simulink subsystem "PEC_LQR"  (R2024a)
settings: Solver=VariableStepAuto  StartTime=0.0  StopTime=10.0  RelTol=1e-3
undefined symbols (not defined in the file): Sim, vehicle
settings Model: Creator=gurt1  LastModifiedBy=gurt1

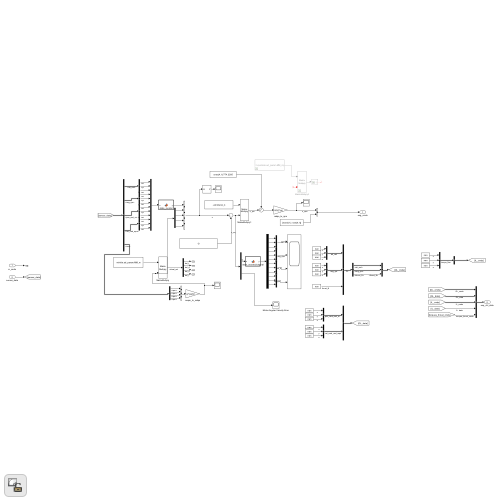
[thumbnail: Simulink's stored preview of the top-level diagram]
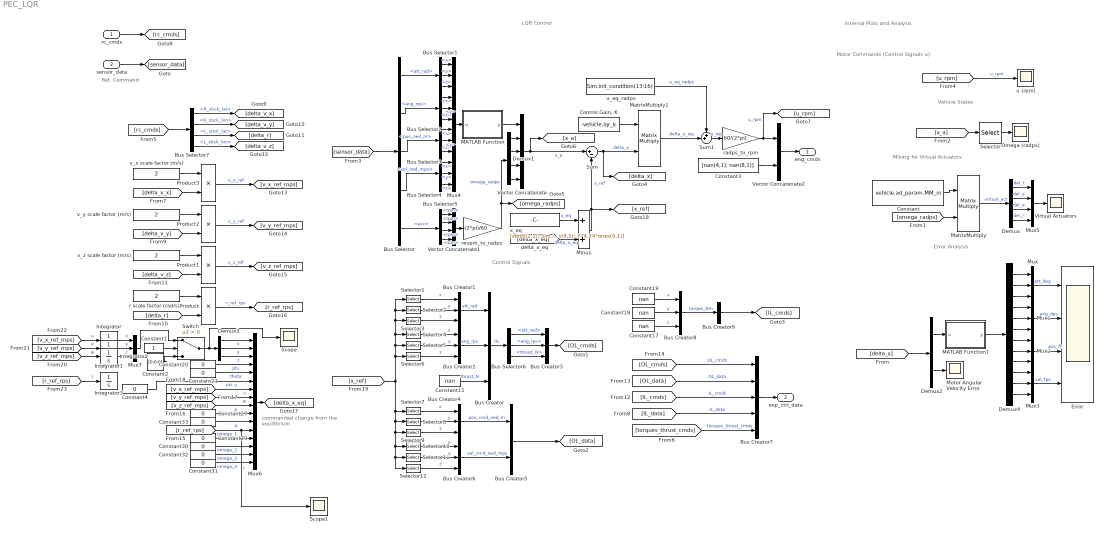
== system PEC_LQR ==
  note: commanded change from the equilibrium
  note: Control Signals
  note: Mixing for Virtual Actuators
  note: Error Analysis
  note: LQR Control
  note: Internal Plots and Analysis
  note: Vehicle States
  note: Motor Commands (Control Signals u)
  note: Ref. Command
  rc_cmds : Inport
  sensor_data : Inport  Port=2
  Bus Creator{,1..4,6,8} (7 alike) : BusCreator  Inputs=3
  Bus Creator5 : BusCreator  Inputs=2
  Bus Creator7 : BusCreator  Inputs=5
  Bus Creator9 : BusCreator  Inputs=1
  Bus Selector : BusSelector  OutputSignals=att_rad,ang_rps,pos_ned_m,vel_ned_mps,esc
  Bus Selector{1..4} (4 alike) : BusSelector  OutputSignals=x,y,z
  Bus Selector5 : BusSelector  OutputSignals=1.rpm,2.rpm,3.rpm,4.rpm
  Bus Selector6 : BusSelector  OutputSignals=att_rad,ang_rps,thrust_N
  Bus Selector7 : BusSelector  OutputSignals=sticks.R_stick_lat,sticks.R_stick_lon,sticks.L_stick_lat,sticks.L_stick_lon
  Constant : Constant  Value=vehicle.ad_param.MM_m
  Constant1 : Constant
  Constant{11,17..19} (4 alike) : Constant  Value=nan
  Constant2 : Constant  Value=[0;0;0]
  Constant{4,20..21,27,29..33} (9 alike) : Constant  Value=0
  Constant3 : Constant  Value=[nan(4,1); nan(8,1)]
  "Control Gain, K" : Constant  Value=-vehicle.lqr_k
  Demux : Demux
  Demux1 : Demux
  Demux2 : Demux  Outputs=[12 4]
  Demux3 : Demux  Outputs=3
  Demux4 : Demux  Outputs=12
  Error : Scope  NumInputPorts=4
  Integrator{,1..3} (4 alike) : Integrator
  MATLAB Function : MATLAB Function  TreatAsAtomicUnit=on
  MATLAB Function1 : MATLAB Function  TreatAsAtomicUnit=on
  MatrixMultiply : Product  Multiplication=Matrix(*)
  MatrixMultiply1 : Product  Multiplication=Matrix(*)
  Minus : Sum
  Motor Angular Velocity Error : Scope
  Mux{,1..3,7} (5 alike) : Mux  Inputs=3
  Mux4 : Mux  Inputs=12
  Mux5 : Mux
  Mux6 : Mux  Inputs=16
  Omega (radps) : Scope
  Product{,1..3} (4 alike) : Product
  Scope : Scope
  Scope1 : Scope
  Selector : Selector  InputPortWidth=16  IndexOptions=Index vector (dialog)  Indices=13:16  OutputSizes=1
  Selector1 : Selector  InputPortWidth=16  IndexOptions=Index vector (dialog)  Indices=4  OutputSizes=1
  Selector10 : Selector  InputPortWidth=16  IndexOptions=Index vector (dialog)  Indices=7  OutputSizes=1
  Selector11 : Selector  InputPortWidth=16  IndexOptions=Index vector (dialog)  Indices=8  OutputSizes=1
  Selector12 : Selector  InputPortWidth=16  IndexOptions=Index vector (dialog)  Indices=9  OutputSizes=1
  Selector2 : Selector  InputPortWidth=16  IndexOptions=Index vector (dialog)  Indices=5  OutputSizes=1
  Selector3 : Selector  InputPortWidth=16  IndexOptions=Index vector (dialog)  Indices=6  OutputSizes=1
  Selector4 : Selector  InputPortWidth=16  IndexOptions=Index vector (dialog)  Indices=10  OutputSizes=1
  Selector5 : Selector  InputPortWidth=16  IndexOptions=Index vector (dialog)  Indices=11  OutputSizes=1
  Selector6 : Selector  InputPortWidth=16  IndexOptions=Index vector (dialog)  Indices=12  OutputSizes=1
  Selector7 : Selector  InputPortWidth=16  IndexOptions=Index vector (dialog)  Indices=1  OutputSizes=1
  Selector8 : Selector  InputPortWidth=16  IndexOptions=Index vector (dialog)  Indices=2  OutputSizes=1
  Selector9 : Selector  InputPortWidth=16  IndexOptions=Index vector (dialog)  Indices=3  OutputSizes=1
  Sum : Sum  Inputs=|+-
  Sum1 : Sum  Inputs=++|
  Switch : Switch  Criteria=u2 > Threshold  SaturateOnIntegerOverflow=off  InputSameDT=off
  Vector Concatenate : Concatenate  NumInputs=5
  Vector Concatenate1 : Concatenate  NumInputs=4
  Vector Concatenate2 : Concatenate
  Virtual Actuators : Scope
  r scale factor (rad/s) : Constant  Value=2
  radps_to_rpm : Gain  Gain=60/(2*pi)
  revpm_to_radps : Gain  Gain=(2*pi)/60
  u (rpm) : Scope
  u_eq_radps : Constant  Value=Sim.init_condition(13:16)
  v_x scale factor (m/s) : Constant  Value=2
  v_y scale factor (m/s) : Constant  Value=2
  v_z scale factor (m/s) : Constant  Value=2
  x_eq : Constant  Value=[zeros(2,1); Sim.init_condition(12);zeros(9,1); 774.24*ones(4,1)]
  eng_cmds : Outport
  exp_ctrl_data : Outport  Port=2
  wires:
  Bus Selector5/4 -> Vector Concatenate1/4  "<rpm>"
  Bus Creator9/1 -> [IL_cmds]
  Selector2/1 -> Bus Creator1/2  "y"
  Demux4/10 -> Mux3/1
  Demux4/8 -> Mux2/2
  Bus Creator4/1 -> Bus Creator5/1  "pos_cmd_ned_m"
  Bus Creator5/1 -> [OL_data]
  Vector Concatenate2/1 -> eng_cmds/1
  Demux4/12 -> Mux3/3
  Selector/1 -> Omega (radps)/1
  Bus Selector/1 -> Bus Selector1/1  "<att_rad>"
  Demux4/6 -> Mux1/3
  u_eq_radps/1 -> Sum1/1  "u_eq_radps"
  Mux/1 -> Error/1  "att_deg"
  Bus Selector6/1 -> Bus Creator3/1  "<att_rad>"
  Bus Selector4/1 -> Mux4/10  "<x>"
  Bus Selector5/1 -> Vector Concatenate1/1  "<rpm>"
  Bus Selector3/1 -> Mux4/7  "<x>"
  Bus Creator1/1 -> Bus Creator/1  "att_rad"
  Bus Selector1/3 -> Mux4/3  "<z>"
  MatrixMultiply/1 -> Demux/1  "virtual_act"
  Vector Concatenate/1 -> [x_a], Sum/1  "x_a"
  Demux4/7 -> Mux2/1
  Selector7/1 -> Bus Creator4/1  "x"
  MatrixMultiply1/1 -> Sum1/2  "delta_u_rps"
  Demux4/9 -> Mux2/3
  Bus Selector/4 -> Bus Selector4/1  "<vel_ned_mps>"
  Selector10/1 -> Bus Creator6/1  "x"
  Selector12/1 -> Bus Creator6/3  "z"
  Demux4/11 -> Mux3/2
  [IL_cmds] -> Bus Creator7/3  "IL_cmds"
  Demux4/2 -> Mux/2
  Constant/1 -> MatrixMultiply/1
  Bus Selector3/3 -> Mux4/9  "<z>"
  "Control Gain, K"/1 -> MatrixMultiply1/1
  Bus Creator6/1 -> Bus Creator5/2  "vel_cmd_ned_mps"
  Constant11/1 -> Bus Creator/3  "thrust_N"
  Bus Selector/2 -> Bus Selector2/1  "<ang_rps>"
  [torques_thrust_cmds] -> Bus Creator7/5  "torques_thrust_cmds"
  Bus Creator2/1 -> Bus Creator/2  "ang_rps"
  Constant18/1 -> Bus Creator8/2  "y"
  Sum1/1 -> radps_to_rpm/1  "u_rps"
  Bus Creator/1 -> Bus Selector6/1  "OL"
  Bus Creator3/1 -> [OL_cmds]
  Bus Selector2/3 -> Mux4/6  "<z>"
  Demux/2 -> Mux5/2  "del_a"
  Constant3/1 -> Vector Concatenate2/2
  Bus Selector5/3 -> Vector Concatenate1/3  "<rpm>"
  Selector8/1 -> Bus Creator4/2  "y"
  [OL_cmds] -> Bus Creator7/1  "OL_cmds"
  Bus Selector/3 -> Bus Selector3/1  "<pos_ned_m>"
  [OL_data] -> Bus Creator7/2  "OL_data"
  x_eq/1 -> Minus/1  "x_eq"
  Demux1/4 -> Vector Concatenate/5
  Selector6/1 -> Bus Creator2/3  "z"
  radps_to_rpm/1 -> Vector Concatenate2/1, [u_rpm]  "u_rpm"
  Selector4/1 -> Bus Creator2/1  "x"
  Bus Selector6/3 -> Bus Creator3/3  "<thrust_N>"
  Selector1/1 -> Bus Creator1/1  "x"
  Bus Selector6/2 -> Bus Creator3/2  "<ang_rps>"
  Sum/1 -> MatrixMultiply1/2, [delta_x]  "delta_x"
  Demux1/3 -> Vector Concatenate/4
  Selector11/1 -> Bus Creator6/2  "y"
  Bus Selector/5 -> Bus Selector5/1  "<esc>"
  Selector5/1 -> Bus Creator2/2  "y"
  Constant19/1 -> Bus Creator8/1  "x"
  Vector Concatenate1/1 -> revpm_to_radps/1
  Bus Creator7/1 -> exp_ctrl_data/1
  Bus Selector1/2 -> Mux4/2  "<y>"
  Bus Creator8/1 -> Bus Creator9/1  "torque_Nm"
  Demux/4 -> Mux5/4  "del_r"
  Mux4/1 -> MATLAB Function/1(u)
  [IL_data] -> Bus Creator7/4  "IL_data"
  Mux1/1 -> Error/2  "ang_dps"
  Mux2/1 -> Error/3  "pos_ft"
  [sensor_data] -> Bus Selector/1
  Bus Selector5/2 -> Vector Concatenate1/2  "<rpm>"
  Mux3/1 -> Error/4  "vel_fps"
  Demux1/2 -> Vector Concatenate/3
  Selector9/1 -> Bus Creator4/3  "z"
  Demux1/1 -> Vector Concatenate/2
  Bus Selector2/1 -> Mux4/4  "<x>"
  Constant17/1 -> Bus Creator8/3  "z"
  Selector3/1 -> Bus Creator1/3  "z"
  MATLAB Function/1(y) -> Vector Concatenate/1
  Bus Selector2/2 -> Mux4/5  "<y>"
  Demux/3 -> Mux5/3  "del_e"
  Bus Selector4/2 -> Mux4/11  "<y>"
  Bus Selector3/2 -> Mux4/8  "<y>"
  Demux2/1 -> MATLAB Function1/1(u)
  Demux2/2 -> Motor Angular Velocity Error/1
  Bus Selector1/1 -> Mux4/1  "<x>"
  Bus Selector4/3 -> Mux4/12  "<z>"
  MATLAB Function1/1(y) -> Demux4/1
  Demux4/1 -> Mux/1
  Demux4/4 -> Mux1/1
  Demux4/3 -> Mux/3
  Demux/1 -> Mux5/1  "del_t"
  Demux4/5 -> Mux1/2
  sensor_data/1 -> [sensor_data]
  rc_cmds/1 -> [rc_cmds]
  [delta_x] -> Demux2/1
  revpm_to_radps/1 -> [omega_radps], Demux1/1  "omega_radps"
  [omega_radps] -> MatrixMultiply/2
  [x_a] -> Selector/1
  Mux5/1 -> Virtual Actuators/1
  [u_rpm] -> u (rpm)/1  "u_rpm"
  [rc_cmds] -> Bus Selector7/1
  Bus Selector7/1 -> [delta_v_x]  "<R_stick_lat>"
  Bus Selector7/4 -> [delta_v_z]  "<L_stick_lon>"
  Bus Selector7/3 -> [delta_r]  "<L_stick_lat>"
  Bus Selector7/2 -> [delta_v_y]  "<R_stick_lon>"
  [delta_r] -> Product/2
  r scale factor (rad/s)/1 -> Product/1
  v_z scale factor (m/s)/1 -> Product1/1
  [delta_v_z] -> Product1/2
  [delta_v_y] -> Product2/2
  v_y scale factor (m/s)/1 -> Product2/1
  [delta_v_x] -> Product3/2
  v_x scale factor (m/s)/1 -> Product3/1
  Product3/1 -> [v_x_ref_mps]  "v_x_ref"
  Product2/1 -> [v_y_ref_mps]  "v_y_ref"
  Product1/1 -> [v_z_ref_mps]  "v_z_ref"
  Product/1 -> [r_ref_rps]  "r_ref_rps"
  Mux6/1 -> [delta_x_eq]
  Demux3/1 -> Mux6/1  "x"
  Demux3/2 -> Mux6/2  "y"
  Demux3/3 -> Mux6/3  "z"
  Constant20/1 -> Mux6/4  "phi"
  Constant21/1 -> Mux6/5  "theta"
  Constant4/1 -> Mux6/6  "psi"
  [v_x_ref_mps] -> Mux6/7  "u"
  [v_z_ref_mps] -> Mux6/9  "w"
  Constant27/1 -> Mux6/10  "p"
  Constant33/1 -> Mux6/11  "q"
  [r_ref_rps] -> Mux6/12, Scope1/1  "r"
  Constant29/1 -> Mux6/13  "omega_1"
  Constant30/1 -> Mux6/14  "omega_2"
  Constant32/1 -> Mux6/15  "omega_3"
  Constant31/1 -> Mux6/16  "omega_4"
  [v_y_ref_mps] -> Mux6/8  "v"
  [delta_x_eq] -> Minus/2  "delta_x_eq"
  Minus/1 -> Sum/2, [x_ref]  "x_ref"
  [x_ref] -> Selector6/1, Selector5/1, Selector1/1, Selector2/1, Selector3/1, Selector4/1, Selector12/1, Selector11/1, Selector10/1, Selector9/1, Selector8/1, Selector7/1
  [v_x_ref_mps] -> Integrator/1  "u"
  [v_y_ref_mps] -> Integrator1/1  "v"
  [v_z_ref_mps] -> Integrator2/1  "w"
  Integrator/1 -> Mux7/1  "x"
  Integrator1/1 -> Mux7/2  "y"
  Integrator2/1 -> Mux7/3  "z"
  Constant1/1 -> Switch/2
  Constant2/1 -> Switch/3
  Mux7/1 -> Switch/1
  Switch/1 -> Demux3/1, Scope/1
  [r_ref_rps] -> Integrator3/1  "r"

== matlab function PEC_LQR/MATLAB Function1 ==
  data: u input; y output
function y = state_reorder2original(u)

    % Transforms from this order: [x, y, z, phi, theta, psi, u, v, w, p, q, r]
    % Back to the original order: [phi, theta, psi, p, q, r, x, y, z, u, v, w]
    
    % Reverse the transformation to the original order
    y = u([4, 5, 6, 10, 11, 12, 1, 2, 3, 7, 8, 9]);

== matlab function PEC_LQR/MATLAB Function ==
  data: u input; y output
function y = state_reorder(u)

% Transforms this: [phi,theta,psi,p,q,r,x,y,z,u,v,w]
% To this order: [x,y,z,phi,theta,psi,u,v,w,p,q,r]
% Transformation to desired order
 y = u([7, 8, 9, 1, 2, 3, 10, 11, 12, 4, 5, 6]);
